simulink model "SF051A_SnsrOffsLrng"  (R2013b)
settings: Solver=FixedStepDiscrete  SolverMode=SingleTasking  StartTime=0.0  StopTime=1  FixedStep=0.002  RelTol=1e-3
undefined symbols (not defined in the file): ARCHGLBPRM_10MILLISEC_SEC_F32, ARCHGLBPRM_2MILLISEC_SEC_F32, ARCHGLBPRM_2PI_ULS_F32, ARCHGLBPRM_FLOATZEROTHD_ULS_F32, ARCHGLBPRM_PIOVER180_ULS_F32, CNV100MICROSECTOMILLISEC_MILLISECPERCNT_F32, CNV100MICROSECTOSEC_SECPERCNT_F32, COVRAMTRXNIT_ULS_F32, HWAUTHYTHD_ULS_F32, HWTQLRNGSTSLRND_CNT_U08, HWTQLRNGSTSNEGOFFS_CNT_U08, HWTQLRNGSTSNOTLRND_CNT_U08, HWTQLRNGSTSPOSOFFS_CNT_U08, HWTQLRNGSTSZEROOFFS_CNT_U08, HWTQLRNGTMRHILIM_SEC_F32, IDYMTRX_ULS_F32, IVS10MS_ULSPERSEC_F32, LRNGFILTICON_ULS_F32, NvmGetErrSts1, ONE_ULS_F32, SnsrOffsLrnd, SnsrOffsLrngFctEna, SnsrOffsLrngHwAgLrngDrvgDstThd, SnsrOffsLrngHwAgLrngEna, SnsrOffsLrngHwAgLrngHwVelThd, SnsrOffsLrngHwAgLrngSysTqThd, SnsrOffsLrngHwAgLrngSysTqThdMed, SnsrOffsLrngHwAgLrngSysTqThdTrustd, SnsrOffsLrngHwAgLrngSysTqThdWide, SnsrOffsLrngHwAgLrngTi, SnsrOffsLrngHwAgLrngVehSpdThd, SnsrOffsLrngHwAgLrngYawOffsDbnd, SnsrOffsLrngHwAgLrngYawRateThd, SnsrOffsLrngHwAgOffsLim, SnsrOffsLrngHwTqLrngEna, SnsrOffsLrngHwTqLrngEnaTiThd, SnsrOffsLrngHwTqLrngHwAgDbnd, SnsrOffsLrngHwTqLrngHwAgThd, SnsrOffsLrngHwTqLrngHwTqThd, SnsrOffsLrngHwTqLrngHwTqZeroOffsThd, SnsrOffsLrngHwTqLrngHwVelThd, SnsrOffsLrngHwTqLrngMeasTi, SnsrOffsLrngHwTqLrngMeasTiScar, SnsrOffsLrngHwTqLrngSampleImbThd1, SnsrOffsLrngHwTqLrngSampleImbThd2, SnsrOffsLrngHwTqLrngSampleThd1, SnsrOffsLrngHwTqLrngSampleThd2, SnsrOffsLrngHwTqLrngTiWghtCoeff, SnsrOffsLrngHwTqLrngVehSpdThd, SnsrOffsLrngHwTqOffsLim, SnsrOffsLrngSampleCntForHwTqLrngRst, SnsrOffsLrngTqInpDetnPwrEstimnThd, SnsrOffsLrngTqInpDetnSinGenrAmp, SnsrOffsLrngTqInpDetnSinGenrFrq, SnsrOffsLrngTqInpDetnStg1FilGain, SnsrOffsLrngTqInpDetnStg1WinSize, SnsrOffsLrngTqInpDetnStg2FilGainCen, SnsrOffsLrngTqInpDetnStg2FilGainDwn, SnsrOffsLrngTqInpDetnStg2FilGainUp, SnsrOffsLrngTqInpDetnStg2WinSize ... (+15)
libraries: Fil x34, FixdToFloat x17, FloatToFixd x16, NxtrLim x15, simulink x12, NxtrAbslt x12, NxtrNvM x8, NxtrMin x5, NxtrMath x3
(part 10 of 11)

== system SF051A_SnsrOffsLrng/SnsrOffsLrng/SnsrOffsLrngPer1/EnableLearning/Perform_TqInpDetn/Enable_PreProcessing/Preprocessing/PrevOut_NoReset ==
  note: Use previous value.
  note: Save loop counter.
  note: Simulink needs to write the number of elapsed loops
      |  here instead of in the Samples counter. Otherwise the
      | write action in the NewOut_ResetCntr action block does not work.
  TqInpDetnPreProcEnaLoop : Inport
  Action Port : ActionPort  ActionType=then
  Data Store Read : DataStoreRead  DataStoreName=TqInpDetnHwTqPreProc
  Data Store Write : DataStoreWrite  DataStoreName=TqInpDetnPreProcEnaLoop
  Subsystem5 : Subsystem  Description=|  mask(Copyright Information){none=on}
      | Copyright info block.                                               
      |                                                                     
      | Place copyright information at the top of every subsystem in design.
      mask prompts: none "No parameters"
      mask help: Place copyright information at the top of every subsystem in design.
      mask Display:
      | NxtrConf = 'Nexteer Confidential';
      | 
      | sys = bdroot; %handle for the current model ("system")
      | first = get_param(sys,'Created');
      | first = first(end-3:end);  %year is last four digits
      | 
      | last = get_param(sys,'LastModifiedDate');
      | if isempty(last)
      |     last = datestr(now,'yyyy');
      | else
      |     last = last(end-3:end);
      | end
      | 
      | if strcmp(first,last)
      |     fprintf('%s -- Copyright %s Nexteer',NxtrConf,first)
      | else
      |     fprintf('%s -- %s%s- %s Nexteer',NxtrConf,char(169),first,last)
      | end
  HwTqPreproc : Outport
  wires:
  Data Store Read/1 -> HwTqPreproc/1
  TqInpDetnPreProcEnaLoop/1 -> Data Store Write/1

== system SF051A_SnsrOffsLrng/SnsrOffsLrng/SnsrOffsLrngPer1/EnableLearning/Perform_TqInpDetn/Enable_PreProcessing/Preprocessing/SampleCounter ==
  note: Limit changed to a Min block.
  HiLim : Inport
  Add : Sum
  Data Store Read : DataStoreRead  DataStoreName=TqInpDetnPreProcEnaLoop
  Min_u16 : NxtrMin/Min_u16  SFunctionSpec=uint16 y1 = Min_u16(uint16 u1, uint16 u2)  ShowSpec=off
      settings: AttributesFormatString=%<Name>
  One_Count : Constant  OutDataTypeStr=uint16
      settings: AttributesFormatString=%<OutDataTypeStr>
  Subsystem5 : Subsystem  Description=|  mask(Copyright Information){none=on}
      | Copyright info block.                                               
      |                                                                     
      | Place copyright information at the top of every subsystem in design.
      mask prompts: none "No parameters"
      mask help: Place copyright information at the top of every subsystem in design.
      mask Display:
      | NxtrConf = 'Nexteer Confidential';
      | 
      | sys = bdroot; %handle for the current model ("system")
      | first = get_param(sys,'Created');
      | first = first(end-3:end);  %year is last four digits
      | 
      | last = get_param(sys,'LastModifiedDate');
      | if isempty(last)
      |     last = datestr(now,'yyyy');
      | else
      |     last = last(end-3:end);
      | end
      | 
      | if strcmp(first,last)
      |     fprintf('%s -- Copyright %s Nexteer',NxtrConf,first)
      | else
      |     fprintf('%s -- %s%s- %s Nexteer',NxtrConf,char(169),first,last)
      | end
  TqInpDetnPreProcEnaLoop : Outport
  wires:
  One_Count/1 -> Add/1
  Data Store Read/1 -> Add/2
  Add/1 -> Min_u16/1
  Min_u16/1 -> TqInpDetnPreProcEnaLoop/1  "TqInpDetnPreProcEnaLoop"
  HiLim/1 -> Min_u16/2

== system SF051A_SnsrOffsLrng/SnsrOffsLrng/SnsrOffsLrngPer1/EnableLearning/Perform_TqInpDetn/Enable_PreProcessing/Preprocessing/Sliding_Goertzel_ver001 ==
  HwTqFild : Inport
  Add : Sum
  SinGen : Subsystem
  SlidingGoertzel : Subsystem
  Subsystem5 : Subsystem  Description=|  mask(Copyright Information){none=on}
      | Copyright info block.                                               
      |                                                                     
      | Place copyright information at the top of every subsystem in design.
      mask prompts: none "No parameters"
      mask help: Place copyright information at the top of every subsystem in design.
      mask Display:
      | NxtrConf = 'Nexteer Confidential';
      | 
      | sys = bdroot; %handle for the current model ("system")
      | first = get_param(sys,'Created');
      | first = first(end-3:end);  %year is last four digits
      | 
      | last = get_param(sys,'LastModifiedDate');
      | if isempty(last)
      |     last = datestr(now,'yyyy');
      | else
      |     last = last(end-3:end);
      | end
      | 
      | if strcmp(first,last)
      |     fprintf('%s -- Copyright %s Nexteer',NxtrConf,first)
      | else
      |     fprintf('%s -- %s%s- %s Nexteer',NxtrConf,char(169),first,last)
      | end
  Stg1Outp : Outport
  wires:
  SinGen/1(TqOscCmd) -> Add/2
  HwTqFild/1 -> Add/1
  SlidingGoertzel/1(Stg1Outp) -> Stg1Outp/1
  Add/1 -> SlidingGoertzel/1(HwTq)

== system SF051A_SnsrOffsLrng/SnsrOffsLrng/SnsrOffsLrngPer1/EnableLearning/Perform_TqInpDetn/Enable_PreProcessing/Preprocessing/Subsystem5 ==

== system SF051A_SnsrOffsLrng/SnsrOffsLrng/SnsrOffsLrngPer1/Learning/ForgettingFactor/ResetHwTqLrng/GetRefTmr100MicroSec32bit/CopyRight2 ==

== system SF051A_SnsrOffsLrng/SnsrOffsLrng/SnsrOffsLrngPer1/Learning/ValidityCheck/DecideOutputs/HwTrqNotLearnt/Subsystem5 ==

== system SF051A_SnsrOffsLrng/SnsrOffsLrng/SnsrOffsLrngPer1/Learning/ValidityCheck/DecideOutputs/HwTrqOffsetLearnt/Subsystem5 ==

== system SF051A_SnsrOffsLrng/SnsrOffsLrng/SnsrOffsLrngPer1/Learning/ValidityCheck/DecideOutputs/Pos//Neg//Zero Offset Status Selector/1_Positive HwTrq Offset ==
  Action Port : ActionPort  ActionType=then
  Constant3 : Constant  Value=HWTQLRNGSTSPOSOFFS_CNT_U08  OutDataTypeStr=uint8
  Subsystem5 : Subsystem  Description=|  mask(Copyright Information){none=on}
      | Copyright info block.                                               
      |                                                                     
      | Place copyright information at the top of every subsystem in design.
      mask prompts: none "No parameters"
      mask help: Place copyright information at the top of every subsystem in design.
      mask Display:
      | NxtrConf = 'Nexteer Confidential';
      | 
      | sys = bdroot; %handle for the current model ("system")
      | first = get_param(sys,'Created');
      | first = first(end-3:end);  %year is last four digits
      | 
      | last = get_param(sys,'LastModifiedDate');
      | if isempty(last)
      |     last = datestr(now,'yyyy');
      | else
      |     last = last(end-3:end);
      | end
      | 
      | if strcmp(first,last)
      |     fprintf('%s -- Copyright %s Nexteer',NxtrConf,first)
      | else
      |     fprintf('%s -- %s%s- %s Nexteer',NxtrConf,char(169),first,last)
      | end
  TOCStatus : Outport
  wires:
  Constant3/1 -> TOCStatus/1

== system SF051A_SnsrOffsLrng/SnsrOffsLrng/SnsrOffsLrngPer1/Learning/ValidityCheck/DecideOutputs/Pos//Neg//Zero Offset Status Selector/2_Negative HwTrq Offset ==
  Action Port : ActionPort  ActionType=elseif
  Constant3 : Constant  Value=HWTQLRNGSTSNEGOFFS_CNT_U08  OutDataTypeStr=uint8
  Subsystem5 : Subsystem  Description=|  mask(Copyright Information){none=on}
      | Copyright info block.                                               
      |                                                                     
      | Place copyright information at the top of every subsystem in design.
      mask prompts: none "No parameters"
      mask help: Place copyright information at the top of every subsystem in design.
      mask Display:
      | NxtrConf = 'Nexteer Confidential';
      | 
      | sys = bdroot; %handle for the current model ("system")
      | first = get_param(sys,'Created');
      | first = first(end-3:end);  %year is last four digits
      | 
      | last = get_param(sys,'LastModifiedDate');
      | if isempty(last)
      |     last = datestr(now,'yyyy');
      | else
      |     last = last(end-3:end);
      | end
      | 
      | if strcmp(first,last)
      |     fprintf('%s -- Copyright %s Nexteer',NxtrConf,first)
      | else
      |     fprintf('%s -- %s%s- %s Nexteer',NxtrConf,char(169),first,last)
      | end
  TOCStatus : Outport
  wires:
  Constant3/1 -> TOCStatus/1

== system SF051A_SnsrOffsLrng/SnsrOffsLrng/SnsrOffsLrngPer1/Learning/ValidityCheck/DecideOutputs/Pos//Neg//Zero Offset Status Selector/3_Zero HwTrq Offset ==
  Action Port : ActionPort  ActionType=else
  Constant3 : Constant  Value=HWTQLRNGSTSZEROOFFS_CNT_U08  OutDataTypeStr=uint8
  Subsystem5 : Subsystem  Description=|  mask(Copyright Information){none=on}
      | Copyright info block.                                               
      |                                                                     
      | Place copyright information at the top of every subsystem in design.
      mask prompts: none "No parameters"
      mask help: Place copyright information at the top of every subsystem in design.
      mask Display:
      | NxtrConf = 'Nexteer Confidential';
      | 
      | sys = bdroot; %handle for the current model ("system")
      | first = get_param(sys,'Created');
      | first = first(end-3:end);  %year is last four digits
      | 
      | last = get_param(sys,'LastModifiedDate');
      | if isempty(last)
      |     last = datestr(now,'yyyy');
      | else
      |     last = last(end-3:end);
      | end
      | 
      | if strcmp(first,last)
      |     fprintf('%s -- Copyright %s Nexteer',NxtrConf,first)
      | else
      |     fprintf('%s -- %s%s- %s Nexteer',NxtrConf,char(169),first,last)
      | end
  TOCStatus : Outport
  wires:
  Constant3/1 -> TOCStatus/1

== system SF051A_SnsrOffsLrng/SnsrOffsLrng/SnsrOffsLrngPer1/Learning/ValidityCheck/DecideOutputs/Pos//Neg//Zero Offset Status Selector/Subsystem5 ==

== system SF051A_SnsrOffsLrng/SnsrOffsLrng/SnsrOffsLrngPer2/Enable_Function/POC/Learn/BiasEstimation_ValidityCheck/Do nothing ==
  Action Port : ActionPort  ActionType=else
  Subsystem1 : Subsystem  Description=|  mask(Copyright Information){none=on}
      | Copyright info block.                                               
      |                                                                     
      | Place copyright information at the top of every subsystem in design.
      mask prompts: none "No parameters"
      mask help: Place copyright information at the top of every subsystem in design.
      mask Display:
      | NxtrConf = 'Nexteer Confidential';
      | 
      | sys = bdroot; %handle for the current model ("system")
      | first = get_param(sys,'Created');
      | first = first(end-3:end);  %year is last four digits
      | 
      | last = get_param(sys,'LastModifiedDate');
      | if isempty(last)
      |     last = datestr(now,'yyyy');
      | else
      |     last = last(end-3:end);
      | end
      | 
      | if strcmp(first,last)
      |     fprintf('%s -- Copyright %s Nexteer',NxtrConf,first)
      | else
      |     fprintf('%s -- %s%s- %s Nexteer',NxtrConf,char(169),first,last)
      | end

== system SF051A_SnsrOffsLrng/SnsrOffsLrng/SnsrOffsLrngPer2/Enable_Function/POC/Learn/BiasEstimation_ValidityCheck/HwTqAvrg_Check ==
  note: Merge blocks changed to 5 inputs.
  note: Case (0) was removed to avoid coverage issues.
      | Signal HwTqLrngSts only gets values between 0 and 4 and the
      | default case was never reached. In this way, default case is
      | reached when HwTqLrngSts is 0 (Content of default block does NOT change).
  note: SysTrq is the addition of the Driver's torque and the Assist torque
      | (in HwNm coordinates)
  note: SysTrqAVG is the average SysTrq during the time that the
      | Learning filters were enabled.
  note: TOCStatus
      | 0 = HwTrq NotLearned
      | 1 = Positive HwTrq Offset
      | 2 = Negative HwTrqOffset
      | 3 = Zero HwTrq Offset
      | 4 = HwTrq Offset Learned
  SysTqAvrg : Inport
  HwTqLrngSts : Inport  Port=2  OutDataTypeStr=uint8
  Constant : Constant  Value=SnsrOffsLrngHwAgLrngSysTqThdTrustd  OutDataTypeStr=single
  Constant1 : Constant  Value=SnsrOffsLrngHwAgLrngSysTqThdWide  OutDataTypeStr=single
  Constant2 : Constant  Value=SnsrOffsLrngHwAgLrngSysTqThdMed  OutDataTypeStr=single
  Display1 : DataStoreWrite  DataStoreName=dSnsrOffsLrngHwAgLrngSysTqUpThd
  Display2 : DataStoreWrite  DataStoreName=dSnsrOffsLrngHwAgLrngSysTqLoThd
  Display3 : DataStoreWrite  DataStoreName=dSnsrOffsLrngHwAgLrngSysTqVldt
  Logical Operator : Logic  AllPortsSameDT=off  OutDataTypeStr=boolean
  Merge_LowTh : Merge  Inputs=5
  Merge_UpTh : Merge  Inputs=5
  Relational Operator : RelationalOperator  Operator=<=  OutDataTypeStr=boolean
  Relational Operator1 : RelationalOperator  OutDataTypeStr=boolean
  Subsystem5 : Subsystem  Description=|  mask(Copyright Information){none=on}
      | Copyright info block.                                               
      |                                                                     
      | Place copyright information at the top of every subsystem in design.
      mask prompts: none "No parameters"
      mask help: Place copyright information at the top of every subsystem in design.
      mask Display:
      | NxtrConf = 'Nexteer Confidential';
      | 
      | sys = bdroot; %handle for the current model ("system")
      | first = get_param(sys,'Created');
      | first = first(end-3:end);  %year is last four digits
      | 
      | last = get_param(sys,'LastModifiedDate');
      | if isempty(last)
      |     last = datestr(now,'yyyy');
      | else
      |     last = last(end-3:end);
      | end
      | 
      | if strcmp(first,last)
      |     fprintf('%s -- Copyright %s Nexteer',NxtrConf,first)
      | else
      |     fprintf('%s -- %s%s- %s Nexteer',NxtrConf,char(169),first,last)
      | end
  Switch Case : SwitchCase  CaseConditions={1,2,3,4}
  Switch Case Action Subsystem1 : Subsystem  RequirementInfo={'linktype_rmi_doors' '0000babd (/E-STEER Core/SubSystem Specifications/Application Functions/SF051A Sensor Offset Learning)' '#SF051A_145' 'true' 'REQ:SF051A_145' '' } %GIDa_07809d37_1ffe_4fb4_b852_393f01c2375c  TreatAsAtomicUnit=on
  Switch Case Action Subsystem2 : Subsystem  RequirementInfo={'linktype_rmi_doors' '0000babd (/E-STEER Core/SubSystem Specifications/Application Functions/SF051A Sensor Offset Learning)' '#SF051A_144' 'true' 'REQ:SF051A_144' '' } %GIDa_dd268c2c_ea11_4446_9a40_dacfc2e25d53  TreatAsAtomicUnit=on
  Switch Case Action Subsystem3 : Subsystem  RequirementInfo={'linktype_rmi_doors' '0000babd (/E-STEER Core/SubSystem Specifications/Application Functions/SF051A Sensor Offset Learning)' '#SF051A_143' 'true' 'REQ:SF051A_143' '' } %GIDa_217b07df_1d8f_435d_a8bd_62cab7965346  TreatAsAtomicUnit=on
  Switch Case Action Subsystem4 : Subsystem  RequirementInfo={'linktype_rmi_doors' '0000babd (/E-STEER Core/SubSystem Specifications/Application Functions/SF051A Sensor Offset Learning)' '#SF051A_142' 'true' 'REQ:SF051A_142' '' } %GIDa_01db2596_4f13_4ac9_b73b_dfc9e16a8861  TreatAsAtomicUnit=on
  Switch Case Action Subsystem5 : Subsystem  TreatAsAtomicUnit=on
  TqVldFlg : Outport
  wires:
  HwTqLrngSts/1 -> Switch Case/1
  Merge_UpTh/1 -> Relational Operator/2, Display1/1
  Merge_LowTh/1 -> Display2/1, Relational Operator1/2
  Switch Case/1 -> Switch Case Action Subsystem1/Action
  Switch Case/2 -> Switch Case Action Subsystem2/Action
  Switch Case/3 -> Switch Case Action Subsystem3/Action
  Switch Case Action Subsystem1/1(UpTh) -> Merge_UpTh/1
  Switch Case Action Subsystem2/1(UpTh) -> Merge_UpTh/2
  Switch Case Action Subsystem3/1(UpTh) -> Merge_UpTh/3
  Switch Case Action Subsystem4/1(UpTh) -> Merge_UpTh/4
  Switch Case Action Subsystem1/2(LowTh) -> Merge_LowTh/1
  Switch Case Action Subsystem2/2(LowTh) -> Merge_LowTh/2
  Switch Case Action Subsystem3/2(LowTh) -> Merge_LowTh/3
  Switch Case Action Subsystem4/2(LowTh) -> Merge_LowTh/4
  Constant1/1 -> Switch Case Action Subsystem2/1(SysTqThdWide), Switch Case Action Subsystem5/1(SysTqThdWide), Switch Case Action Subsystem1/1(SysTqThdWide)
  Constant/1 -> Switch Case Action Subsystem4/1(SysTqThdTrustd)
  Constant2/1 -> Switch Case Action Subsystem3/1(SysTqThdMed)
  Switch Case/5 -> Switch Case Action Subsystem5/Action
  Switch Case Action Subsystem5/1(UpTh) -> Merge_UpTh/5
  Switch Case Action Subsystem5/2(LowTh) -> Merge_LowTh/5
  SysTqAvrg/1 -> Relational Operator/1, Relational Operator1/1
  Relational Operator/1 -> Logical Operator/1
  Logical Operator/1 -> Display3/1, TqVldFlg/1
  Relational Operator1/1 -> Logical Operator/2
  Switch Case/4 -> Switch Case Action Subsystem4/Action

== system SF051A_SnsrOffsLrng/SnsrOffsLrng/SnsrOffsLrngPer2/Enable_Function/POC/Learn/BiasEstimation_ValidityCheck/Keep OR Reset ==
  note: The function learned for long enough, but the average (slowly filtered)
      | system torque was excessive, indicating road crown, cross wind, etc.
  HwPosBiasEstRaw : Inport
  TqVldFlg : Inport  Port=2
  Action Port : ActionPort  ActionType=then
  If2 : If  IfExpression=u1
  Limit and Keep Learned Value : Subsystem  RequirementInfo={'linktype_rmi_doors' '0000babd (/E-STEER Core/SubSystem Specifications/Application Functions/SF051A Sensor Offset Learning)' '#SF051A_141' 'true' 'REQ:SF051A_141' '' } %GIDa_1f0e41ab_d12e_487c_96e6_f1739bc149ed  TreatAsAtomicUnit=on
  Reset_HwAgLrng : Subsystem  TreatAsAtomicUnit=on
  Subsystem5 : Subsystem  Description=|  mask(Copyright Information){none=on}
      | Copyright info block.                                               
      |                                                                     
      | Place copyright information at the top of every subsystem in design.
      mask prompts: none "No parameters"
      mask help: Place copyright information at the top of every subsystem in design.
      mask Display:
      | NxtrConf = 'Nexteer Confidential';
      | 
      | sys = bdroot; %handle for the current model ("system")
      | first = get_param(sys,'Created');
      | first = first(end-3:end);  %year is last four digits
      | 
      | last = get_param(sys,'LastModifiedDate');
      | if isempty(last)
      |     last = datestr(now,'yyyy');
      | else
      |     last = last(end-3:end);
      | end
      | 
      | if strcmp(first,last)
      |     fprintf('%s -- Copyright %s Nexteer',NxtrConf,first)
      | else
      |     fprintf('%s -- %s%s- %s Nexteer',NxtrConf,char(169),first,last)
      | end
  wires:
  TqVldFlg/1 -> If2/1
  HwPosBiasEstRaw/1 -> Limit and Keep Learned Value/1(HwPosBiasEstRaw)
  If2/1 -> Limit and Keep Learned Value/Action
  If2/2 -> Reset_HwAgLrng/Action

== system SF051A_SnsrOffsLrng/SnsrOffsLrng/SnsrOffsLrngPer2/Enable_Function/POC/Learn/BiasEstimation_ValidityCheck/Subsystem5 ==

== system SF051A_SnsrOffsLrng/SnsrOffsLrng/SnsrOffsLrngPer2/Enable_Function/POC/Learn/BiasEstimation_ValidityCheck/Time_Check ==
  note: Limit changed to a Min block. Code might not be affected.
  ElpsdTi : Inport  RequirementInfo={'linktype_rmi_doors' '0000babd (/E-STEER Core/SubSystem Specifications/Application Functions/SF051A Sensor Offset Learning)' '#SF051A_118' 'true' 'REQ:SF051A_118' '' } %GIDa_ec54a004_f423_4b2c_b946_d1b5b6921296
  Constant1 : Constant  RequirementInfo={'linktype_rmi_doors' '0000babd (/E-STEER Core/SubSystem Specifications/Application Functions/SF051A Sensor Offset Learning)' '#SF051A_122' 'true' 'REQ:SF051A_122' '' ; 'linktype_rmi_doors' '0000babd (/E-STEER Core/SubSystem Specifications/Application Functions/SF051A Sensor Offset Learning)' '#SF051A_117' 'true' 'REQ:SF051A_117' '' } %GIDa_c643d9d6_48fd_4a4d_910f_6142205684cf  Value=SnsrOffsLrngHwAgLrngTi
  Constant2 : Constant  RequirementInfo={'linktype_rmi_doors' '0000babd (/E-STEER Core/SubSystem Specifications/Application Functions/SF051A Sensor Offset Learning)' '#SF051A_122' 'true' 'REQ:SF051A_122' '' ; 'linktype_rmi_doors' '0000babd (/E-STEER Core/SubSystem Specifications/Application Functions/SF051A Sensor Offset Learning)' '#SF051A_117' 'true' 'REQ:SF051A_117' '' } %GIDa_4f74e54b_b333_4f57_8398_1a745c9dd038  Value=SnsrOffsLrngHwAgLrngTi
  Display1 : DataStoreWrite  DataStoreName=dSnsrOffsLrngHwAgLrngTiVldt
  Min_f32 : NxtrMin/Min_f32  SFunctionSpec=single y1 = Min_f32(single u1, single u2)
      settings: AttributesFormatString=%<Name>
  Relational Operator1 : RelationalOperator  RequirementInfo={'linktype_rmi_doors' '0000babd (/E-STEER Core/SubSystem Specifications/Application Functions/SF051A Sensor Offset Learning)' '#SF051A_117' 'true' 'REQ:SF051A_117' '' } %GIDa_e756bea4_804a_407e_bb48_f5c0006da0a9  OutDataTypeStr=boolean
  Subsystem5 : Subsystem  Description=|  mask(Copyright Information){none=on}
      | Copyright info block.                                               
      |                                                                     
      | Place copyright information at the top of every subsystem in design.
      mask prompts: none "No parameters"
      mask help: Place copyright information at the top of every subsystem in design.
      mask Display:
      | NxtrConf = 'Nexteer Confidential';
      | 
      | sys = bdroot; %handle for the current model ("system")
      | first = get_param(sys,'Created');
      | first = first(end-3:end);  %year is last four digits
      | 
      | last = get_param(sys,'LastModifiedDate');
      | if isempty(last)
      |     last = datestr(now,'yyyy');
      | else
      |     last = last(end-3:end);
      | end
      | 
      | if strcmp(first,last)
      |     fprintf('%s -- Copyright %s Nexteer',NxtrConf,first)
      | else
      |     fprintf('%s -- %s%s- %s Nexteer',NxtrConf,char(169),first,last)
      | end
  Write NVMRam : DataStoreWrite  RequirementInfo={'linktype_rmi_doors' '0000babd (/E-STEER Core/SubSystem Specifications/Application Functions/SF051A Sensor Offset Learning)' '#SF051A_120' 'true' 'REQ:SF051A_120' '' ; 'linktype_rmi_doors' '0000babd (/E-STEER Core/SubSystem Specifications/Application Functions/SF051A Sensor Offset Learning)' '#SF051A_119' 'true' 'REQ:SF051A_119' '' ; 'linktype_rmi_doors' '0000babd (/E-STEER Core/SubSystem Specifications/Application Functions/SF051A Sensor Offset Learning)' '#SF051A_118' 'true' 'REQ:SF051A_118' '' } %GIDa_6fdf401b_98e4_4250_8664_c2ed6dbc601a  DataStoreName=SnsrOffsLrnd  DataStoreElements=SnsrOffsLrnd.HwAgLrndTi
  TiVldFlg : Outport
  wires:
  ElpsdTi/1 -> Min_f32/1, Relational Operator1/1  "ElpsdTi"
  Min_f32/1 -> Write NVMRam/1
  Constant1/1 -> Relational Operator1/2
  Relational Operator1/1 -> Display1/1, TiVldFlg/1
  Constant2/1 -> Min_f32/2

== system SF051A_SnsrOffsLrng/SnsrOffsLrng/SnsrOffsLrngPer2/Enable_Function/POC/Learn/LPFs/Subsystem5 ==

== system SF051A_SnsrOffsLrng/SnsrOffsLrng/SnsrOffsLrngPer2/Enable_Function/POC/Learning Conditions/DrivingStraight/Subsystem5 ==

== system SF051A_SnsrOffsLrng/SnsrOffsLrng/SnsrOffsLrngPer2/Enable_Function/POC/Learning Conditions/NotDrivingStraight/Subsystem5 ==

== system SF051A_SnsrOffsLrng/SnsrOffsLrng/SnsrOffsLrngPer2/Enable_Function/YOC/Learn/Do nothing/Subsystem5 ==

== system SF051A_SnsrOffsLrng/SnsrOffsLrng/SnsrOffsLrngPer2/Enable_Function/YOC/Learn/Filter For Learning/Subsystem5 ==

== system SF051A_SnsrOffsLrng/SnsrOffsLrng/SnsrOffsLrngPer2/Enable_Function/YOC/Learn/Update NVM RAM/Subsystem5 ==

== system SF051A_SnsrOffsLrng/SnsrOffsLrng/SnsrOffsLrngPer1/EnableLearning/Perform_TqInpDetn/Enable_PreProcessing/If Action Subsystem/True_False/Subsystem5 ==

== system SF051A_SnsrOffsLrng/SnsrOffsLrng/SnsrOffsLrngPer1/EnableLearning/Perform_TqInpDetn/Enable_PreProcessing/If Action Subsystem/True_True/Subsystem5 ==

== system SF051A_SnsrOffsLrng/SnsrOffsLrng/SnsrOffsLrngPer1/EnableLearning/Perform_TqInpDetn/Enable_PreProcessing/Preprocessing/Do nothing/Subsystem5 ==

== system SF051A_SnsrOffsLrng/SnsrOffsLrng/SnsrOffsLrngPer1/EnableLearning/Perform_TqInpDetn/Enable_PreProcessing/Preprocessing/General_Goertzel/Goertzel_Part1_1 ==
  note: s(n-2)
  note: Suggested Coding:  This can be an inline local function.  Simulink limitations prevent modeling it that way, so this block
      | is replicated multiple times throughout the component model.
  X0 : Inport
  FilGain : Inport  Port=2
  S2 : Inport  Port=3
  S1 : Inport  Port=4
  " Product1" : Product  Inputs=**
  Add1 : Sum  Inputs=++-
  Subsystem5 : Subsystem  Description=|  mask(Copyright Information){none=on}
      | Copyright info block.                                               
      |                                                                     
      | Place copyright information at the top of every subsystem in design.
      mask prompts: none "No parameters"
      mask help: Place copyright information at the top of every subsystem in design.
      mask Display:
      | NxtrConf = 'Nexteer Confidential';
      | 
      | sys = bdroot; %handle for the current model ("system")
      | first = get_param(sys,'Created');
      | first = first(end-3:end);  %year is last four digits
      | 
      | last = get_param(sys,'LastModifiedDate');
      | if isempty(last)
      |     last = datestr(now,'yyyy');
      | else
      |     last = last(end-3:end);
      | end
      | 
      | if strcmp(first,last)
      |     fprintf('%s -- Copyright %s Nexteer',NxtrConf,first)
      | else
      |     fprintf('%s -- %s%s- %s Nexteer',NxtrConf,char(169),first,last)
      | end
  S0 : Outport
  wires:
  Add1/1 -> S0/1
  " Product1"/1 -> Add1/2
  S2/1 -> Add1/3
  FilGain/1 -> " Product1"/1
  X0/1 -> Add1/1
  S1/1 -> " Product1"/2

== system SF051A_SnsrOffsLrng/SnsrOffsLrng/SnsrOffsLrngPer1/EnableLearning/Perform_TqInpDetn/Enable_PreProcessing/Preprocessing/General_Goertzel/Goertzel_Part1_2 ==
  note: s(n-2)
  note: Suggested Coding:  This can be an inline local function.  Simulink limitations prevent modeling it that way, so this block
      | is replicated multiple times throughout the component model.
  X0 : Inport
  FilGain : Inport  Port=2
  S2 : Inport  Port=3
  S1 : Inport  Port=4
  " Product1" : Product  Inputs=**
  Add1 : Sum  Inputs=++-
  Subsystem5 : Subsystem  Description=|  mask(Copyright Information){none=on}
      | Copyright info block.                                               
      |                                                                     
      | Place copyright information at the top of every subsystem in design.
      mask prompts: none "No parameters"
      mask help: Place copyright information at the top of every subsystem in design.
      mask Display:
      | NxtrConf = 'Nexteer Confidential';
      | 
      | sys = bdroot; %handle for the current model ("system")
      | first = get_param(sys,'Created');
      | first = first(end-3:end);  %year is last four digits
      | 
      | last = get_param(sys,'LastModifiedDate');
      | if isempty(last)
      |     last = datestr(now,'yyyy');
      | else
      |     last = last(end-3:end);
      | end
      | 
      | if strcmp(first,last)
      |     fprintf('%s -- Copyright %s Nexteer',NxtrConf,first)
      | else
      |     fprintf('%s -- %s%s- %s Nexteer',NxtrConf,char(169),first,last)
      | end
  S0 : Outport
  wires:
  Add1/1 -> S0/1
  " Product1"/1 -> Add1/2
  S2/1 -> Add1/3
  FilGain/1 -> " Product1"/1
  X0/1 -> Add1/1
  S1/1 -> " Product1"/2

== system SF051A_SnsrOffsLrng/SnsrOffsLrng/SnsrOffsLrngPer1/EnableLearning/Perform_TqInpDetn/Enable_PreProcessing/Preprocessing/General_Goertzel/Goertzel_Part1_3 ==
  note: s(n-2)
  note: Suggested Coding:  This can be an inline local function.  Simulink limitations prevent modeling it that way, so this block
      | is replicated multiple times throughout the component model.
  X0 : Inport
  FilGain : Inport  Port=2
  S2 : Inport  Port=3
  S1 : Inport  Port=4
  " Product1" : Product  Inputs=**
  Add1 : Sum  Inputs=++-
  Subsystem5 : Subsystem  Description=|  mask(Copyright Information){none=on}
      | Copyright info block.                                               
      |                                                                     
      | Place copyright information at the top of every subsystem in design.
      mask prompts: none "No parameters"
      mask help: Place copyright information at the top of every subsystem in design.
      mask Display:
      | NxtrConf = 'Nexteer Confidential';
      | 
      | sys = bdroot; %handle for the current model ("system")
      | first = get_param(sys,'Created');
      | first = first(end-3:end);  %year is last four digits
      | 
      | last = get_param(sys,'LastModifiedDate');
      | if isempty(last)
      |     last = datestr(now,'yyyy');
      | else
      |     last = last(end-3:end);
      | end
      | 
      | if strcmp(first,last)
      |     fprintf('%s -- Copyright %s Nexteer',NxtrConf,first)
      | else
      |     fprintf('%s -- %s%s- %s Nexteer',NxtrConf,char(169),first,last)
      | end
  S0 : Outport
  wires:
  Add1/1 -> S0/1
  " Product1"/1 -> Add1/2
  S2/1 -> Add1/3
  FilGain/1 -> " Product1"/1
  X0/1 -> Add1/1
  S1/1 -> " Product1"/2

== system SF051A_SnsrOffsLrng/SnsrOffsLrng/SnsrOffsLrngPer1/EnableLearning/Perform_TqInpDetn/Enable_PreProcessing/Preprocessing/General_Goertzel/Subsystem5 ==

== system SF051A_SnsrOffsLrng/SnsrOffsLrng/SnsrOffsLrngPer1/EnableLearning/Perform_TqInpDetn/Enable_PreProcessing/Preprocessing/NewOut_ResetCntr/Goertzel_Part2_1 ==
  note: abs(y(n))^2
  note: Suggested Coding:  This can be an inline local function.  Simulink limitations prevent modeling it that way, so this block
      | is replicated multiple times throughout the component model.
  note: s^2(n)
  note: s^2(n-1)
  note: s(n-1)
  note: In the academic definition of the goertzel algorithm this block would have a complex calculation.
      | Since we are only interested in the magnitude, the following is an implementation that only need real calculations.
  S0 : Inport
  S1 : Inport  Port=2
  FilGain : Inport  Port=3
  " Product5" : Product  Inputs=**
  Product2 : Product  Inputs=**
  Product3 : Product  Inputs=**
  Product4 : Product  Inputs=**
  Subsystem5 : Subsystem  Description=|  mask(Copyright Information){none=on}
      | Copyright info block.                                               
      |                                                                     
      | Place copyright information at the top of every subsystem in design.
      mask prompts: none "No parameters"
      mask help: Place copyright information at the top of every subsystem in design.
      mask Display:
      | NxtrConf = 'Nexteer Confidential';
      | 
      | sys = bdroot; %handle for the current model ("system")
      | first = get_param(sys,'Created');
      | first = first(end-3:end);  %year is last four digits
      | 
      | last = get_param(sys,'LastModifiedDate');
      | if isempty(last)
      |     last = datestr(now,'yyyy');
      | else
      |     last = last(end-3:end);
      | end
      | 
      | if strcmp(first,last)
      |     fprintf('%s -- Copyright %s Nexteer',NxtrConf,first)
      | else
      |     fprintf('%s -- %s%s- %s Nexteer',NxtrConf,char(169),first,last)
      | end
  add : Sum  Inputs=++-
  MagnSq : Outport
  wires:
  FilGain/1 -> " Product5"/2
  add/1 -> MagnSq/1
  Product2/1 -> add/1  "FiltSt0Sq_Uls_T_f32"
  Product3/1 -> add/2  "FiltSt1Sq_Uls_T_f32"
  Product4/1 -> " Product5"/1
  " Product5"/1 -> add/3  "FiltSt0St1_Uls_T_f32"
  S1/1 -> Product3/2, Product3/1, Product4/2
  S0/1 -> Product4/1, Product2/2, Product2/1

== system SF051A_SnsrOffsLrng/SnsrOffsLrng/SnsrOffsLrngPer1/EnableLearning/Perform_TqInpDetn/Enable_PreProcessing/Preprocessing/NewOut_ResetCntr/Goertzel_Part2_2 ==
  note: abs(y(n))^2
  note: Suggested Coding:  This can be an inline local function.  Simulink limitations prevent modeling it that way, so this block
      | is replicated multiple times throughout the component model.
  note: s^2(n)
  note: s^2(n-1)
  note: s(n-1)
  note: In the academic definition of the goertzel algorithm this block would have a complex calculation.
      | Since we are only interested in the magnitude, the following is an implementation that only need real calculations.
  S0 : Inport
  S1 : Inport  Port=2
  FilGain : Inport  Port=3
  " Product5" : Product  Inputs=**
  Product2 : Product  Inputs=**
  Product3 : Product  Inputs=**
  Product4 : Product  Inputs=**
  Subsystem5 : Subsystem  Description=|  mask(Copyright Information){none=on}
      | Copyright info block.                                               
      |                                                                     
      | Place copyright information at the top of every subsystem in design.
      mask prompts: none "No parameters"
      mask help: Place copyright information at the top of every subsystem in design.
      mask Display:
      | NxtrConf = 'Nexteer Confidential';
      | 
      | sys = bdroot; %handle for the current model ("system")
      | first = get_param(sys,'Created');
      | first = first(end-3:end);  %year is last four digits
      | 
      | last = get_param(sys,'LastModifiedDate');
      | if isempty(last)
      |     last = datestr(now,'yyyy');
      | else
      |     last = last(end-3:end);
      | end
      | 
      | if strcmp(first,last)
      |     fprintf('%s -- Copyright %s Nexteer',NxtrConf,first)
      | else
      |     fprintf('%s -- %s%s- %s Nexteer',NxtrConf,char(169),first,last)
      | end
  add : Sum  Inputs=++-
  MagnSq : Outport
  wires:
  FilGain/1 -> " Product5"/2
  add/1 -> MagnSq/1
  Product2/1 -> add/1  "FiltSt0Sq_Uls_T_f32"
  Product3/1 -> add/2  "FiltSt1Sq_Uls_T_f32"
  Product4/1 -> " Product5"/1
  " Product5"/1 -> add/3  "FiltSt0St1_Uls_T_f32"
  S1/1 -> Product3/2, Product3/1, Product4/2
  S0/1 -> Product4/1, Product2/2, Product2/1

== system SF051A_SnsrOffsLrng/SnsrOffsLrng/SnsrOffsLrngPer1/EnableLearning/Perform_TqInpDetn/Enable_PreProcessing/Preprocessing/NewOut_ResetCntr/Goertzel_Part2_3 ==
  note: abs(y(n))^2
  note: Suggested Coding:  This can be an inline local function.  Simulink limitations prevent modeling it that way, so this block
      | is replicated multiple times throughout the component model.
  note: s^2(n)
  note: s^2(n-1)
  note: s(n-1)
  note: In the academic definition of the goertzel algorithm this block would have a complex calculation.
      | Since we are only interested in the magnitude, the following is an implementation that only need real calculations.
  S0 : Inport
  S1 : Inport  Port=2
  FilGain : Inport  Port=3
  " Product5" : Product  Inputs=**
  Product2 : Product  Inputs=**
  Product3 : Product  Inputs=**
  Product4 : Product  Inputs=**
  Subsystem5 : Subsystem  Description=|  mask(Copyright Information){none=on}
      | Copyright info block.                                               
      |                                                                     
      | Place copyright information at the top of every subsystem in design.
      mask prompts: none "No parameters"
      mask help: Place copyright information at the top of every subsystem in design.
      mask Display:
      | NxtrConf = 'Nexteer Confidential';
      | 
      | sys = bdroot; %handle for the current model ("system")
      | first = get_param(sys,'Created');
      | first = first(end-3:end);  %year is last four digits
      | 
      | last = get_param(sys,'LastModifiedDate');
      | if isempty(last)
      |     last = datestr(now,'yyyy');
      | else
      |     last = last(end-3:end);
      | end
      | 
      | if strcmp(first,last)
      |     fprintf('%s -- Copyright %s Nexteer',NxtrConf,first)
      | else
      |     fprintf('%s -- %s%s- %s Nexteer',NxtrConf,char(169),first,last)
      | end
  add : Sum  Inputs=++-
  MagnSq : Outport
  wires:
  FilGain/1 -> " Product5"/2
  add/1 -> MagnSq/1
  Product2/1 -> add/1  "FiltSt0Sq_Uls_T_f32"
  Product3/1 -> add/2  "FiltSt1Sq_Uls_T_f32"
  Product4/1 -> " Product5"/1
  " Product5"/1 -> add/3  "FiltSt0St1_Uls_T_f32"
  S1/1 -> Product3/2, Product3/1, Product4/2
  S0/1 -> Product4/1, Product2/2, Product2/1

== system SF051A_SnsrOffsLrng/SnsrOffsLrng/SnsrOffsLrngPer1/EnableLearning/Perform_TqInpDetn/Enable_PreProcessing/Preprocessing/NewOut_ResetCntr/Subsystem5 ==

== system SF051A_SnsrOffsLrng/SnsrOffsLrng/SnsrOffsLrngPer1/EnableLearning/Perform_TqInpDetn/Enable_PreProcessing/Preprocessing/PrevOut_NoReset/Subsystem5 ==

== system SF051A_SnsrOffsLrng/SnsrOffsLrng/SnsrOffsLrngPer1/EnableLearning/Perform_TqInpDetn/Enable_PreProcessing/Preprocessing/SampleCounter/Subsystem5 ==

== system SF051A_SnsrOffsLrng/SnsrOffsLrng/SnsrOffsLrngPer1/EnableLearning/Perform_TqInpDetn/Enable_PreProcessing/Preprocessing/Sliding_Goertzel_ver001/SinGen ==
  note: This generates a sinusoidal command for a given frequency and fixed amplitude.  Based on logic found in SF043A, but simplified because
      | the frequency and amplitude values are just calibrations for this component.
  Add : Sum
  Angle_Wrapper : Subsystem
  Constant : Constant  Value=SnsrOffsLrngTqInpDetnSinGenrFrq
  Constant4 : Constant  Value=SnsrOffsLrngTqInpDetnSinGenrAmp
  Convert_To_Radians : Subsystem  TreatAsAtomicUnit=on
  Data Store Read : DataStoreRead  DataStoreName=TqInpDetnSinGenrAg
  Data Store Write : DataStoreWrite  DataStoreName=TqInpDetnSinGenrAg
  Product2 : Product  OutDataTypeStr=single  RndMeth=Zero
  Sin_f32 : NxtrMath/Sin_f32  SFunctionSpec=single y1 = Sin_f32(single u1)
      settings: AttributesFormatString=%<MaskType>
  Subsystem5 : Subsystem  Description=|  mask(Copyright Information){none=on}
      | Copyright info block.                                               
      |                                                                     
      | Place copyright information at the top of every subsystem in design.
      mask prompts: none "No parameters"
      mask help: Place copyright information at the top of every subsystem in design.
      mask Display:
      | NxtrConf = 'Nexteer Confidential';
      | 
      | sys = bdroot; %handle for the current model ("system")
      | first = get_param(sys,'Created');
      | first = first(end-3:end);  %year is last four digits
      | 
      | last = get_param(sys,'LastModifiedDate');
      | if isempty(last)
      |     last = datestr(now,'yyyy');
      | else
      |     last = last(end-3:end);
      | end
      | 
      | if strcmp(first,last)
      |     fprintf('%s -- Copyright %s Nexteer',NxtrConf,first)
      | else
      |     fprintf('%s -- %s%s- %s Nexteer',NxtrConf,char(169),first,last)
      | end
  TqOscCmd : Outport
  wires:
  Sin_f32/1 -> Product2/2
  Product2/1 -> TqOscCmd/1
  Angle_Wrapper/1(AgOut) -> Sin_f32/1, Data Store Write/1
  Add/1 -> Angle_Wrapper/1(AgIn)
  Constant4/1 -> Product2/1
  Constant/1 -> Convert_To_Radians/1(Freq)
  Convert_To_Radians/1(PhaAgStep) -> Add/1
  Data Store Read/1 -> Add/2

== system SF051A_SnsrOffsLrng/SnsrOffsLrng/SnsrOffsLrngPer1/EnableLearning/Perform_TqInpDetn/Enable_PreProcessing/Preprocessing/Sliding_Goertzel_ver001/SlidingGoertzel ==
  note: Limit to prevent log(0) = -inf
  note: Conversion to dB
  note: NOTE: Cal.EngMin = 1 to prevent divide-by-zero.
  HwTq : Inport
  Calculate_Magnitude : Subsystem
  Constant1 : Constant  Value=SnsrOffsLrngTqInpDetnStg1WinSize
  Constant2 : Constant  Value=TQINPDETNLOGGAIN_ULS_F32
  Data Type Conversion : DataTypeConversion  OutDataTypeStr=single
  Divide : Product  Inputs=*/
  LimStat_f32 : NxtrLim/LimStat_f32  LoLim=TQINPDETNLOGINPLOLIM_ULS_F32  HiLim=TQINPDETNLOGINPHILIM_ULS_F32
      settings: AttributesFormatString=|
      | Low Limit: %<LoLim>
      | High Limit:%<HiLim>
  Math Function1 : Math  Operator=log10  OutputSignalType=real  SaturateOnIntegerOverflow=on
  Product : Product
  Product1 : Product
  Sliding_Input : Subsystem
  Subsystem5 : Subsystem  Description=|  mask(Copyright Information){none=on}
      | Copyright info block.                                               
      |                                                                     
      | Place copyright information at the top of every subsystem in design.
      mask prompts: none "No parameters"
      mask help: Place copyright information at the top of every subsystem in design.
      mask Display:
      | NxtrConf = 'Nexteer Confidential';
      | 
      | sys = bdroot; %handle for the current model ("system")
      | first = get_param(sys,'Created');
      | first = first(end-3:end);  %year is last four digits
      | 
      | last = get_param(sys,'LastModifiedDate');
      | if isempty(last)
      |     last = datestr(now,'yyyy');
      | else
      |     last = last(end-3:end);
      | end
      | 
      | if strcmp(first,last)
      |     fprintf('%s -- Copyright %s Nexteer',NxtrConf,first)
      | else
      |     fprintf('%s -- %s%s- %s Nexteer',NxtrConf,char(169),first,last)
      | end
  Stg1Outp : Outport
  wires:
  Math Function1/1 -> Product1/1
  Product1/1 -> Stg1Outp/1
  HwTq/1 -> Sliding_Input/1(HwTq)
  Sliding_Input/1(x_n) -> Calculate_Magnitude/1(x_n)
  Calculate_Magnitude/1(MgnSq) -> Divide/1
  Product/1 -> Data Type Conversion/1
  Divide/1 -> LimStat_f32/1
  Constant1/1 -> Product/2, Product/1
  Data Type Conversion/1 -> Divide/2
  Constant2/1 -> Product1/2
  LimStat_f32/1 -> Math Function1/1

== system SF051A_SnsrOffsLrng/SnsrOffsLrng/SnsrOffsLrngPer1/EnableLearning/Perform_TqInpDetn/Enable_PreProcessing/Preprocessing/Sliding_Goertzel_ver001/Subsystem5 ==

== system SF051A_SnsrOffsLrng/SnsrOffsLrng/SnsrOffsLrngPer1/Learning/ValidityCheck/DecideOutputs/Pos//Neg//Zero Offset Status Selector/1_Positive HwTrq Offset/Subsystem5 ==

== system SF051A_SnsrOffsLrng/SnsrOffsLrng/SnsrOffsLrngPer1/Learning/ValidityCheck/DecideOutputs/Pos//Neg//Zero Offset Status Selector/2_Negative HwTrq Offset/Subsystem5 ==

== system SF051A_SnsrOffsLrng/SnsrOffsLrng/SnsrOffsLrngPer1/Learning/ValidityCheck/DecideOutputs/Pos//Neg//Zero Offset Status Selector/3_Zero HwTrq Offset/Subsystem5 ==

== system SF051A_SnsrOffsLrng/SnsrOffsLrng/SnsrOffsLrngPer2/Enable_Function/POC/Learn/BiasEstimation_ValidityCheck/Do nothing/Subsystem1 ==

== system SF051A_SnsrOffsLrng/SnsrOffsLrng/SnsrOffsLrngPer2/Enable_Function/POC/Learn/BiasEstimation_ValidityCheck/HwTqAvrg_Check/Subsystem5 ==

== system SF051A_SnsrOffsLrng/SnsrOffsLrng/SnsrOffsLrngPer2/Enable_Function/POC/Learn/BiasEstimation_ValidityCheck/HwTqAvrg_Check/Switch Case Action Subsystem1 ==
  SysTqThdWide : Inport
  Action Port : ActionPort  ActionType=case
  Constant : Constant  Value=ZERO_ULS_F32  OutDataTypeStr=single
      settings: AttributesFormatString=%<OutDataTypeStr>
  Subsystem5 : Subsystem  Description=|  mask(Copyright Information){none=on}
      | Copyright info block.                                               
      |                                                                     
      | Place copyright information at the top of every subsystem in design.
      mask prompts: none "No parameters"
      mask help: Place copyright information at the top of every subsystem in design.
      mask Display:
      | NxtrConf = 'Nexteer Confidential';
      | 
      | sys = bdroot; %handle for the current model ("system")
      | first = get_param(sys,'Created');
      | first = first(end-3:end);  %year is last four digits
      | 
      | last = get_param(sys,'LastModifiedDate');
      | if isempty(last)
      |     last = datestr(now,'yyyy');
      | else
      |     last = last(end-3:end);
      | end
      | 
      | if strcmp(first,last)
      |     fprintf('%s -- Copyright %s Nexteer',NxtrConf,first)
      | else
      |     fprintf('%s -- %s%s- %s Nexteer',NxtrConf,char(169),first,last)
      | end
  UpTh : Outport
  LowTh : Outport  Port=2
  wires:
  SysTqThdWide/1 -> UpTh/1
  Constant/1 -> LowTh/1

== system SF051A_SnsrOffsLrng/SnsrOffsLrng/SnsrOffsLrngPer2/Enable_Function/POC/Learn/BiasEstimation_ValidityCheck/HwTqAvrg_Check/Switch Case Action Subsystem2 ==
  SysTqThdWide : Inport
  Action Port : ActionPort  ActionType=case
  Constant : Constant  Value=ZERO_ULS_F32  OutDataTypeStr=single
      settings: AttributesFormatString=%<OutDataTypeStr>
  Gain : Gain  Gain=-1
  Subsystem5 : Subsystem  Description=|  mask(Copyright Information){none=on}
      | Copyright info block.                                               
      |                                                                     
      | Place copyright information at the top of every subsystem in design.
      mask prompts: none "No parameters"
      mask help: Place copyright information at the top of every subsystem in design.
      mask Display:
      | NxtrConf = 'Nexteer Confidential';
      | 
      | sys = bdroot; %handle for the current model ("system")
      | first = get_param(sys,'Created');
      | first = first(end-3:end);  %year is last four digits
      | 
      | last = get_param(sys,'LastModifiedDate');
      | if isempty(last)
      |     last = datestr(now,'yyyy');
      | else
      |     last = last(end-3:end);
      | end
      | 
      | if strcmp(first,last)
      |     fprintf('%s -- Copyright %s Nexteer',NxtrConf,first)
      | else
      |     fprintf('%s -- %s%s- %s Nexteer',NxtrConf,char(169),first,last)
      | end
  UpTh : Outport
  LowTh : Outport  Port=2
  wires:
  SysTqThdWide/1 -> Gain/1
  Gain/1 -> LowTh/1
  Constant/1 -> UpTh/1

== system SF051A_SnsrOffsLrng/SnsrOffsLrng/SnsrOffsLrngPer2/Enable_Function/POC/Learn/BiasEstimation_ValidityCheck/HwTqAvrg_Check/Switch Case Action Subsystem3 ==
  SysTqThdMed : Inport
  Action Port : ActionPort  ActionType=case
  Gain1 : Gain  Gain=-1
  Subsystem5 : Subsystem  Description=|  mask(Copyright Information){none=on}
      | Copyright info block.                                               
      |                                                                     
      | Place copyright information at the top of every subsystem in design.
      mask prompts: none "No parameters"
      mask help: Place copyright information at the top of every subsystem in design.
      mask Display:
      | NxtrConf = 'Nexteer Confidential';
      | 
      | sys = bdroot; %handle for the current model ("system")
      | first = get_param(sys,'Created');
      | first = first(end-3:end);  %year is last four digits
      | 
      | last = get_param(sys,'LastModifiedDate');
      | if isempty(last)
      |     last = datestr(now,'yyyy');
      | else
      |     last = last(end-3:end);
      | end
      | 
      | if strcmp(first,last)
      |     fprintf('%s -- Copyright %s Nexteer',NxtrConf,first)
      | else
      |     fprintf('%s -- %s%s- %s Nexteer',NxtrConf,char(169),first,last)
      | end
  UpTh : Outport
  LowTh : Outport  Port=2
  wires:
  Gain1/1 -> LowTh/1
  SysTqThdMed/1 -> Gain1/1, UpTh/1
